simulink model "Leds"  (R2023b)
settings: Solver=VariableStepAuto  StartTime=0.0  StopTime=inf  RelTol=1e-3
libraries: arduinolib x3, simulink x1
settings Model: PacingRate=0.100000  Creator=TESTER  LastModifiedBy=TESTER

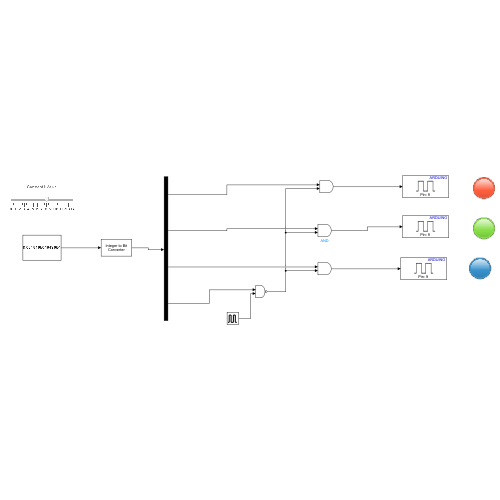
[thumbnail: Simulink's stored preview of the top-level diagram]
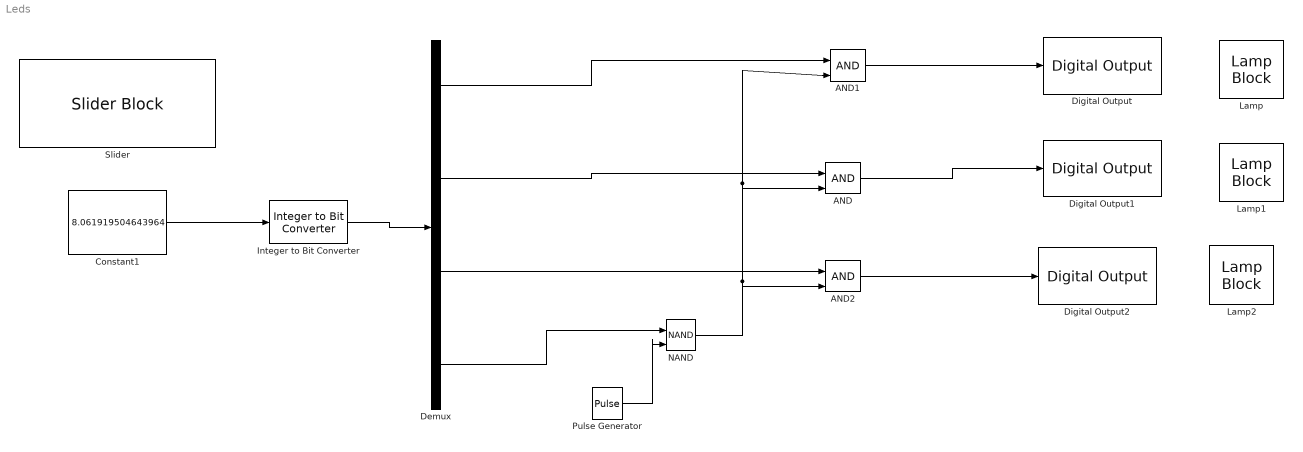
== system Leds ==
  AND : Logic  IconShape=distinctive  AllPortsSameDT=off  OutDataTypeStr=boolean
  AND1 : Logic  IconShape=distinctive  AllPortsSameDT=off  OutDataTypeStr=boolean
  AND2 : Logic  IconShape=distinctive  AllPortsSameDT=off  OutDataTypeStr=boolean
  Constant1 : Constant  Value=8.061919504643964
  Demux : Demux
  Digital Output : arduinolib/Digital Output  pinNumber=9  Direction=output  blockPlatform=arduino
  Digital Output1 : arduinolib/Digital Output  pinNumber=9  Direction=output  blockPlatform=arduino
  Digital Output2 : arduinolib/Digital Output  pinNumber=9  Direction=output  blockPlatform=arduino
  Integer to Bit Converter : simulink/Logic and Bit Operations/Integer to Bit Converter  nbits=4  signedInputValues=Unsigned  bitOrder=MSB first  outDtype=Inherit via internal rule
  Lamp : LampBlock  LabelPosition=Hide
  Lamp1 : LampBlock  LabelPosition=Hide
  Lamp2 : LampBlock  LabelPosition=Hide
  NAND : Logic  Operator=NAND  IconShape=distinctive  AllPortsSameDT=off  OutDataTypeStr=boolean
  Pulse Generator : DiscretePulseGenerator  PulseType=Time based  Period=1  PulseWidth=50
  Slider : SliderBlock  ScaleMax=14  TickInterval=1
  wires:
  AND1/1 -> Digital Output/1
  AND/1 -> Digital Output1/1
  AND2/1 -> Digital Output2/1
  Pulse Generator/1 -> NAND/2
  NAND/1 -> AND2/2, AND1/2, AND/2
  Demux/2 -> AND/1
  Demux/1 -> AND1/1
  Constant1/1 -> Integer to Bit Converter/1
  Integer to Bit Converter/1 -> Demux/1
  Demux/3 -> AND2/1
  Demux/4 -> NAND/1
